simulink model "sim9"  (R2013b)
settings: Solver=ode45  StartTime=0.0  StopTime=10.0  RelTol=1e-3
undefined symbols (not defined in the file or in its folder): i
libraries: commrandsrc2 x5, commdigbbndpm3 x3, commdigbbndam3 x1, commdigbbndfm2 x1
settings Model: Creator=Kseniya  LastModifiedBy=Kseniya

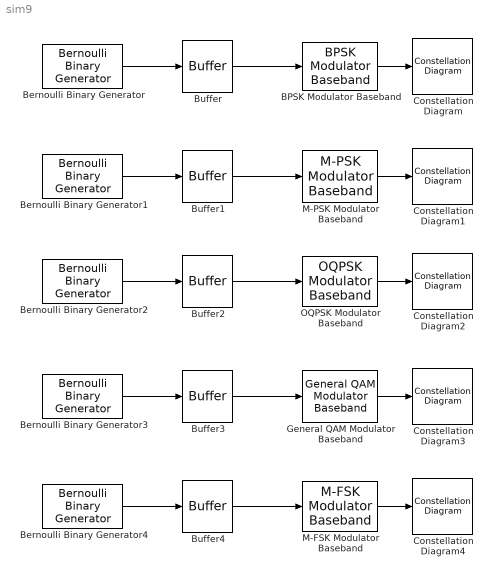
== system sim9 ==
  BPSK Modulator Baseband : commdigbbndpm3/BPSK Modulator Baseband  Ph=0  outDtype=double  outWordLen=16  outUDDataType=sfix(16)  outFracLenMode=Best precision  outFracLen=15
  Bernoulli Binary Generator{,1..4} (5 alike) : commrandsrc2/Bernoulli Binary Generator  P=0.5  seed=61  Ts=1/100  frameBased=off  sampPerFrame=1  orient=off  outDataType=double
  Buffer{,1..4} (5 alike) : Buffer  TreatMby1Signals=One channel
  Constellation Diagram{,1..4} (5 alike) : ConstellationDiagram
      settings: CopyFcn=scopeextensions.ScopeBlock.onCoreBlockCopy(gcbh);  DeleteFcn=scopeextensions.ScopeBlock.callback(gcbh, 'onBlockDelete');  PreSaveFcn=scopeextensions.ScopeBlock.callback(gcbh, 'onModelSave');  NameChangeFcn=scopeextensions.ScopeBlock.callback(gcbh, 'onBlockRename');  DestroyFcn=scopeextensions.ScopeBlock.onBlockDestroy(gcbh)  CloseFcn=scopeextensions.ScopeBlock.callback(gcbh, 'onBlockClose');  PreDeleteFcn=scopeextensions.ScopeBlock.callback(gcbh, 'onBlockPreDelete');
  General QAM Modulator Baseband : commdigbbndam3/General QAM Modulator Baseband  SigCon=[exp(2*pi*i*[0:7]/8)]  outDtype=double  outWordLen=16  outUDDataType=sfix(16)  outFracLenMode=Best precision  outFracLen=15
  M-FSK Modulator Baseband : commdigbbndfm2/M-FSK Modulator Baseband  M=8  InType=Integer  Enc=Gray  freqSep=6  phaseType=Continuous  numSamp=17  RateOptions=Enforce single-rate processing  outDataType=double
  M-PSK Modulator Baseband : commdigbbndpm3/M-PSK Modulator Baseband  M=8  InType=Integer  Enc=Gray  Mapping=[0:7]  Ph=pi/8  outDtype=double  outWordLen=16  outUDDataType=sfix(16)  outFracLenMode=Best precision  outFracLen=15
  OQPSK Modulator Baseband : commdigbbndpm3/OQPSK Modulator Baseband  InType=Integer  Ph=0  RateOptions=Enforce single-rate processing  outDtype=double  outWordLen=16  outUDDataType=sfix(16)  outFracLenMode=Best precision  outFracLen=15
  wires:
  Bernoulli Binary Generator/1 -> Buffer/1
  Buffer/1 -> BPSK Modulator Baseband/1
  BPSK Modulator Baseband/1 -> Constellation Diagram/1
  Bernoulli Binary Generator1/1 -> Buffer1/1
  Buffer1/1 -> M-PSK Modulator Baseband/1
  M-PSK Modulator Baseband/1 -> Constellation Diagram1/1
  Bernoulli Binary Generator2/1 -> Buffer2/1
  Buffer2/1 -> OQPSK Modulator Baseband/1
  OQPSK Modulator Baseband/1 -> Constellation Diagram2/1
  Bernoulli Binary Generator3/1 -> Buffer3/1
  Buffer3/1 -> General QAM Modulator Baseband/1
  General QAM Modulator Baseband/1 -> Constellation Diagram3/1
  Bernoulli Binary Generator4/1 -> Buffer4/1
  Buffer4/1 -> M-FSK Modulator Baseband/1
  M-FSK Modulator Baseband/1 -> Constellation Diagram4/1
